simulink model "EMI_Resilient_Actuator_Phase2B"  (R2026a)
settings: Solver=FixedStepDiscrete  StopTime=1.5  FixedStep=0.001
model workspace (MAT data in the model file):
  EMIActuatorModelSchema.id = 'EMI-ACTUATOR-PARAMETERIZED-V2'
  EMIActuatorModelSchema.kind = 'phase2b'
  EMIActuatorModelSchema.plantInputCount = 2
  EMIActuatorModelSchema.supplyLogColumns = 4
settings Model: Creator=adand  LastModifiedBy=adand

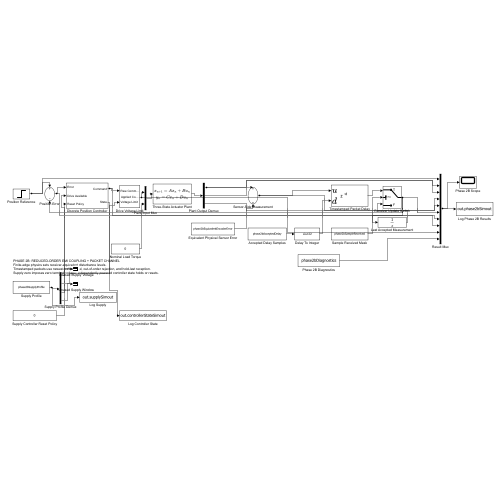
[thumbnail: Simulink's stored preview of the top-level diagram]
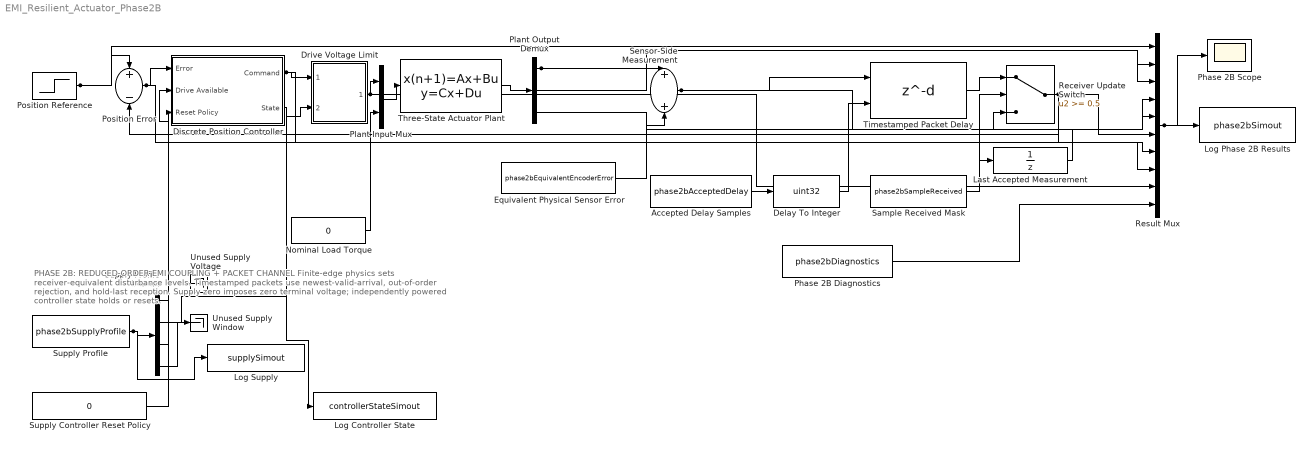
== system EMI_Resilient_Actuator_Phase2B ==
  note: PHASE 2B: REDUCED-ORDER EMI COUPLING + PACKET CHANNEL
      | Finite-edge physics sets receiver-equivalent disturbance levels.
      | Timestamped packets use newest-valid-arrival, out-of-order rejection, and hold-last reception.
      | Supply zero imposes zero terminal voltage; independently powered controller state holds or resets.
  Accepted Delay Samples : FromWorkspace  VariableName=phase2bAcceptedDelay  Interpolate=off  OutputAfterFinalValue=Holding final value
  Delay To Integer : DataTypeConversion  OutDataTypeStr=uint32  SaturateOnIntegerOverflow=off  RndMeth=Floor
  Discrete Position Controller : Subsystem
  Drive Voltage Limit : Subsystem
  Equivalent Physical Sensor Error : FromWorkspace  VariableName=phase2bEquivalentEncoderError  Interpolate=off  OutputAfterFinalValue=Holding final value
  Last Accepted Measurement : UnitDelay  SampleTime=0.001
  Log Controller State : ToWorkspace  VariableName=controllerStateSimout  SaveFormat=Structure With Time  SampleTime=-1
  Log Phase 2B Results : ToWorkspace  VariableName=phase2bSimout  SaveFormat=Structure With Time  SampleTime=-1
  Log Supply : ToWorkspace  VariableName=supplySimout  SaveFormat=Structure With Time  SampleTime=-1
  Nominal Load Torque : Constant  Value=0
  Phase 2B Diagnostics : FromWorkspace  VariableName=phase2bDiagnostics  Interpolate=off  OutputAfterFinalValue=Holding final value
  Phase 2B Scope : Scope
  Plant Input Mux : Mux  Inputs=2
  Plant Output Demux : Demux  Outputs=3
  Position Error : Sum  Inputs=+-
  Position Reference : Step  Time=0.10000000000000001  FinalValue=0.52359877559829882  SampleTime=0.001
  Receiver Update Switch : Switch  Threshold=0.5  SaturateOnIntegerOverflow=off  InputSameDT=off
  Result Mux : Mux  Inputs=10
  Sample Received Mask : FromWorkspace  VariableName=phase2bSampleReceived  Interpolate=off  OutputAfterFinalValue=Holding final value
  Sensor-Side Measurement : Sum
  Supply Controller Reset Policy : Constant  Value=0
  Supply Profile : FromWorkspace  VariableName=phase2bSupplyProfile  Interpolate=off  OutputAfterFinalValue=Holding final value
  Supply Profile Demux : Demux
  Three-State Actuator Plant : DiscreteStateSpace  A=[1 0.0009971362516155032 0.00022829831371848575;0 0.99202969645993144 0.42222281027672853;0 -0.025333368616603714 0.61255694572372166]  B=[3.1636509108574085e-05 -0.0033282765581096828;0.09131932548739434 -6.6475750107700211;0.31678125686440572 0.091319325487394326]  C=[1 0 0;0 1 0;0 0 1]  D=[0 0;0 0;0 0]  InitialCondition=zeros(3,1)  SampleTime=0.001
  Timestamped Packet Delay : Delay  DelayLengthSource=Input port  DelayLengthUpperLimit=16  InitialCondition=0  DiagnosticForDelayLength=Error  SampleTime=0.001
      settings: InputPortMap=u0,p1
  Unused Supply Voltage : Terminator
  Unused Supply Window : Terminator
  wires:
  Position Reference/1 -> Position Error/1, Result Mux/1
  Position Error/1 -> Discrete Position Controller/1(Error), Result Mux/7
  Discrete Position Controller/1(Command) -> Drive Voltage Limit/1(Raw Command), Result Mux/8
  Drive Voltage Limit/1(Applied Command) -> Plant Input Mux/1, Result Mux/9
  Nominal Load Torque/1 -> Plant Input Mux/2
  Plant Input Mux/1 -> Three-State Actuator Plant/1
  Supply Profile/1 -> Supply Profile Demux/1, Log Supply/1
  Supply Profile Demux/1 -> Unused Supply Voltage/1
  Supply Profile Demux/2 -> Drive Voltage Limit/2(Voltage Limit)
  Supply Profile Demux/3 -> Discrete Position Controller/2(Drive Available)
  Supply Profile Demux/4 -> Unused Supply Window/1
  Supply Controller Reset Policy/1 -> Discrete Position Controller/3(Reset Policy)
  Discrete Position Controller/2(State) -> Log Controller State/1
  Three-State Actuator Plant/1 -> Plant Output Demux/1
  Plant Output Demux/1 -> Sensor-Side Measurement/1, Result Mux/2
  Equivalent Physical Sensor Error/1 -> Sensor-Side Measurement/2
  Sensor-Side Measurement/1 -> Timestamped Packet Delay/1, Result Mux/5
  Accepted Delay Samples/1 -> Delay To Integer/1
  Delay To Integer/1 -> Timestamped Packet Delay/2
  Timestamped Packet Delay/1 -> Receiver Update Switch/1
  Sample Received Mask/1 -> Receiver Update Switch/2
  Last Accepted Measurement/1 -> Receiver Update Switch/3
  Receiver Update Switch/1 -> Last Accepted Measurement/1, Position Error/2, Result Mux/6
  Plant Output Demux/2 -> Result Mux/3
  Plant Output Demux/3 -> Result Mux/4
  Phase 2B Diagnostics/1 -> Result Mux/10
  Result Mux/1 -> Phase 2B Scope/1, Log Phase 2B Results/1

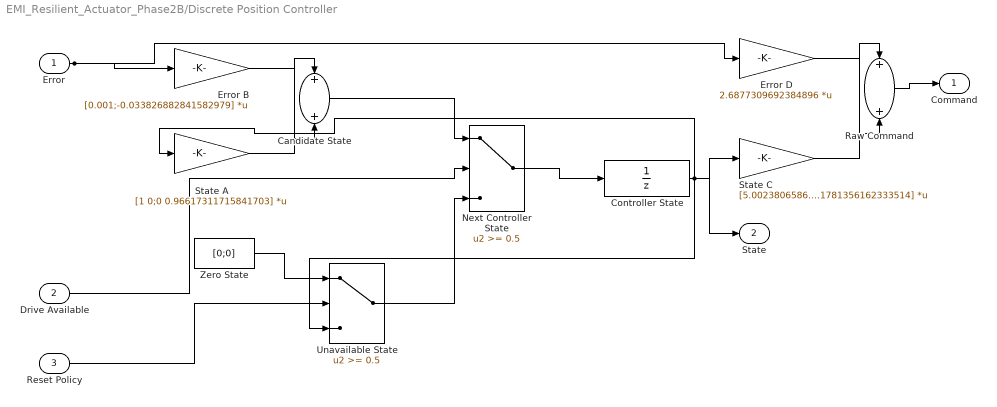
== system EMI_Resilient_Actuator_Phase2B/Discrete Position Controller ==
  Error : Inport
  Drive Available : Inport  Port=2
  Reset Policy : Inport  Port=3
  Candidate State : Sum
  Controller State : UnitDelay  InitialCondition=[0;0]  SampleTime=0.001
  Error B : Gain  Gain=[0.001;-0.033826882841582979]  Multiplication=Matrix(K*u)
  Error D : Gain  Gain=2.6877309692384896  Multiplication=Matrix(K*u)
  Next Controller State : Switch  Threshold=0.5  SaturateOnIntegerOverflow=off  InputSameDT=off
  Raw Command : Sum
  State A : Gain  Gain=[1 0;0 0.96617311715841703]  Multiplication=Matrix(K*u)
  State C : Gain  Gain=[5.0023806586276089 1.1781356162333514]  Multiplication=Matrix(K*u)
  Unavailable State : Switch  Threshold=0.5  SaturateOnIntegerOverflow=off  InputSameDT=off
  Zero State : Constant  Value=[0;0]
  Command : Outport
  State : Outport  Port=2
  wires:
  Error/1 -> Error B/1, Error D/1
  Controller State/1 -> State A/1, State C/1, State/1, Unavailable State/3
  State A/1 -> Candidate State/1
  Error B/1 -> Candidate State/2
  State C/1 -> Raw Command/1
  Error D/1 -> Raw Command/2
  Raw Command/1 -> Command/1
  Zero State/1 -> Unavailable State/1
  Reset Policy/1 -> Unavailable State/2
  Candidate State/1 -> Next Controller State/1
  Drive Available/1 -> Next Controller State/2
  Unavailable State/1 -> Next Controller State/3
  Next Controller State/1 -> Controller State/1

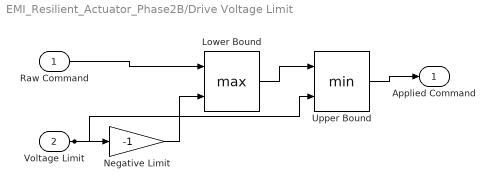
== system EMI_Resilient_Actuator_Phase2B/Drive Voltage Limit ==
  Raw Command : Inport
  Voltage Limit : Inport  Port=2
  Lower Bound : MinMax  Function=max  Inputs=2
  Negative Limit : Gain  Gain=-1
  Upper Bound : MinMax  Inputs=2
  Applied Command : Outport
  wires:
  Raw Command/1 -> Lower Bound/1
  Voltage Limit/1 -> Negative Limit/1, Upper Bound/2
  Negative Limit/1 -> Lower Bound/2
  Lower Bound/1 -> Upper Bound/1
  Upper Bound/1 -> Applied Command/1
